simulink subsystem "Grid_Power_Controller"  (R2021b)
settings: Solver=VariableStepAuto  StartTime=0.0  StopTime=10.0  RelTol=1e-3
model mask{Tavg=gsc.Tavg, Vmag=gsc.Vmag, Ilim=gsc.Ilim, Prated=gsc.Prated, Vdc_nom=ess.Vdc_0, Vdc_del=ess.Vdc_del, kp_v=gsc.kp, ki_v=gsc.ki}
  mask prompts: Tavg "Averaging Time Constant (s):"; Vmag "Grid voltage magnitude (V):"; Ilim "GSC current limit (A):"; Prated "GSC rated power (W):"; Vdc_nom "DC link nominal voltage (V):"; Vdc_del "DC link voltage deviation maximum (V):"; kp_v "Voltage regulator proportional gain:"; ki_v "Voltage regulator integral gain:"
undefined symbols (not defined in the file): simu
libraries: simulink x1
settings Model: Creator=Derek  LastModifiedBy=Derek

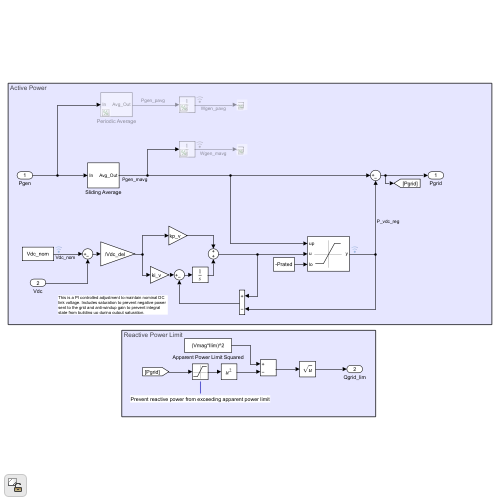
[thumbnail: Simulink's stored preview of the top-level diagram]
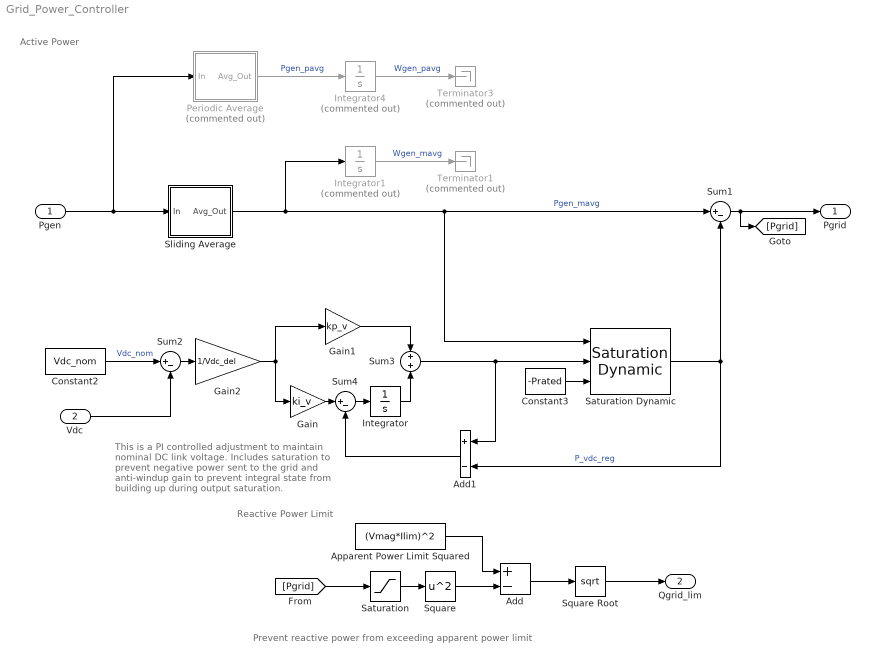
== system Grid_Power_Controller ==
  note: This is a PI controlled adjustment to maintain nominal DC link voltage. Includes saturation to prevent negative power sent to the grid and anti-windup gain to prevent integral state from building up during output saturation.
  note: Reactive Power Limit
  note: Active Power
  note: Prevent reactive power from exceeding apparent power limit
  Pgen : Inport
  Vdc : Inport  Port=2
  Add : Sum  Inputs=+-
  Add1 : Sum  Inputs=+-
  Apparent Power Limit Squared : Constant  Value=(Vmag*Ilim)^2
  Constant2 : Constant  Value=Vdc_nom
  Constant3 : Constant  Value=-Prated
  Gain : Gain  Gain=ki_v
  Gain1 : Gain  Gain=kp_v
  Gain2 : Gain  Gain=1/Vdc_del
  Integrator : Integrator
  Integrator1 : Integrator  Commented=on
  Integrator4 : Integrator  Commented=on
  Periodic Average : Subsystem  Commented=on  mask{Tsample=Tavg}
      mask prompts: Tsample "Sampling Period (s):"
  Saturation : Saturate  UpperLimit=Vmag*Ilim  LowerLimit=-Vmag*Ilim
  Saturation Dynamic : simulink/Discontinuities/Saturation Dynamic  OutMin=[]  OutMax=[]  OutDataTypeStr=Inherit: Same as second input  OutDataType=fixdt(1, 16)  OutScaling=2^-10  DoSatur=off
  Sliding Average : Subsystem  mask{Tsample=Tavg, dt=simu.dt}
      mask prompts: Tsample "Sampling Period (s):"; dt "Simulation Time Step (s):"
  Square : Math  Operator=square  SaturateOnIntegerOverflow=on
  Square Root : Sqrt  SaturateOnIntegerOverflow=on
  Sum1 : Sum  Inputs=|+-
  Sum2 : Sum  Inputs=|+-
  Sum3 : Sum
  Sum4 : Sum  Inputs=|+-
  Terminator1 : Terminator  Commented=on
  Terminator3 : Terminator  Commented=on
  Pgrid : Outport
  Qgrid_lim : Outport  Port=2
  wires:
  Pgen/1 -> Sliding Average/1(In), Periodic Average/1(In)
  Integrator4/1 -> Terminator3/1  "Wgen_pavg"
  Integrator1/1 -> Terminator1/1  "Wgen_mavg"
  Sliding Average/1(Avg_Out) -> Integrator1/1, Sum1/1, Saturation Dynamic/1  "Pgen_mavg"
  Periodic Average/1(Avg_Out) -> Integrator4/1  "Pgen_pavg"
  Add/1 -> Square Root/1
  Square/1 -> Add/2
  Saturation/1 -> Square/1
  Square Root/1 -> Qgrid_lim/1
  Apparent Power Limit Squared/1 -> Add/1
  Sum1/1 -> Pgrid/1, [Pgrid]
  [Pgrid] -> Saturation/1
  Constant2/1 -> Sum2/1  "Vdc_nom"
  Constant3/1 -> Saturation Dynamic/3
  Sum3/1 -> Saturation Dynamic/2, Add1/1
  Gain1/1 -> Sum3/1
  Integrator/1 -> Sum3/2
  Saturation Dynamic/1 -> Sum1/2, Add1/2  "P_vdc_reg"
  Vdc/1 -> Sum2/2
  Sum2/1 -> Gain2/1
  Gain2/1 -> Gain/1, Gain1/1
  Gain/1 -> Sum4/1
  Sum4/1 -> Integrator/1
  Add1/1 -> Sum4/2

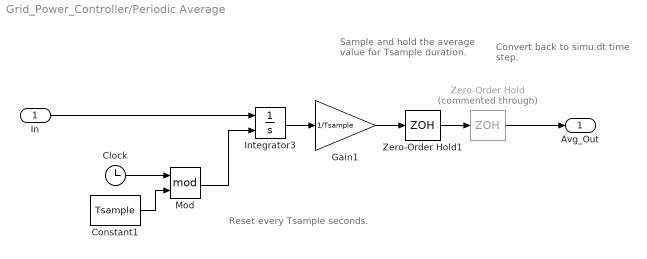
== system Grid_Power_Controller/Periodic Average ==
  note: Sample and hold the average value for Tsample duration.
  note: Convert back to simu.dt time step.
  note: Reset every Tsample seconds.
  In : Inport
  Clock : Clock
  Constant1 : Constant  Value=Tsample
  Gain1 : Gain  Gain=1/Tsample
  Integrator3 : Integrator  ExternalReset=rising
  Mod : Math  Operator=mod  OutputSignalType=real  SaturateOnIntegerOverflow=on
  Zero-Order Hold : ZeroOrderHold  Commented=through  SampleTime=simu.dt
  Zero-Order Hold1 : ZeroOrderHold  SampleTime=Tsample
  Avg_Out : Outport
  wires:
  Constant1/1 -> Mod/2
  In/1 -> Integrator3/1
  Integrator3/1 -> Gain1/1
  Gain1/1 -> Zero-Order Hold1/1
  Clock/1 -> Mod/1
  Zero-Order Hold1/1 -> Zero-Order Hold/1
  Mod/1 -> Integrator3/2
  Zero-Order Hold/1 -> Avg_Out/1

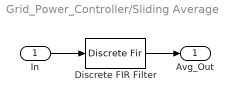
== system Grid_Power_Controller/Sliding Average ==
  In : Inport
  Discrete FIR Filter : DiscreteFir  Coefficients=ones(1,round(Tsample/dt))/round(Tsample/dt)  SampleTime=dt
  Avg_Out : Outport
  wires:
  Discrete FIR Filter/1 -> Avg_Out/1
  In/1 -> Discrete FIR Filter/1
